simulink model "Simulador"  (R2015a)
settings: Solver=ode45  StartTime=0.0  StopTime=Inf  MaxStep=1  RelTol=1e-3
StopFcn:
  | close all
  | post_simulacion
model workspace (MAT data in the model file):
  m = 3.797
  b = 2.1
  c = 0.3571
  Salar = 0.75
  AR = 5.88
  cg = [0.44 0 0]
  Ix = 1.229
  Iy = 0.1702
  Iz = 0.8808
  Ixz = 0.9343
  e = 0.9935
  alpha0 = 0.267
  coefprop = [0.016415 -0.0142726]
  C_L0 = 0.0254
  C_Lalpha = 4.0191
  C_Lq = 3.8954
  C_Ldelta_e = 0.5872
  C_D0 = 0.0102
  C_Dbeta1 = -2.0864e-07
  C_Dbeta2 = 0.0671
  C_Dq = 0
  C_Ddelta_e = 0.8461
  C_Y0 = 3.2049e-18
  C_Ybeta = -0.1949
  C_Yp = -0.1172
  C_Yr = 0.0959
  C_Ydelta_a = -0.0696
  C_l0 = 1.1518e-18
  C_lbeta = -0.0765
  C_lp = -0.4018
  C_lr = 0.025
  C_ldelta_a = 0.2987
  C_m0 = 0.018
  C_malpha = -0.2524
  C_mq = -1.3047
  C_mdelta_e = -0.4857
  C_n0 = -2.2667e-07
  C_nbeta = 0.0403
  C_np = -0.0247
  C_nr = -0.1252
  C_ndelta_a = 0.0076
  gamma = 0.20958671
  gamma1 = 8.64638926772
  gamma2 = 7.15127867602
  gamma3 = 4.20255654569
  gamma4 = 4.4578208227
  gamma5 = -2.04582843713
  gamma6 = 5.48942420682
  gamma7 = 10.3736620037
  gamma8 = 5.86392142899
  C_p0 = -1.01045424588e-06
  C_pbeta = -0.14184539659
  C_pp = -1.79869539438
  C_pr = -0.45305525336
  C_pdelta_a = 1.28918307845
  C_r0 = -1.3291750703e-06
  C_rbeta = -0.104707259349
  C_rp = -1.93599126586
  C_rr = -0.622717442342
  C_rdelta_a = 1.3761168826
  C_mp = -0.2168
values from neighbouring files (symbols this model uses):
  r = [r_n;r_e;r_d]    [segmento.m]
  waypoints = reshape(waypoints_mat.',[],1)    [plan_de_vuelo.m]
undefined symbols (not defined in the file or in its folder): F, Light, magnitude, MIL, plan_de_vuelo
libraries: simulink_extras x20, aerolibconvert2 x18, aerolibfltsims x2, simulink x2, vrlib x1, instrumentlib x1, aerolibatmos2 x1, aerolibtransform2 x1, aerolibwind2 x1, aerolibgravity2 x1
(part 2 of 3)

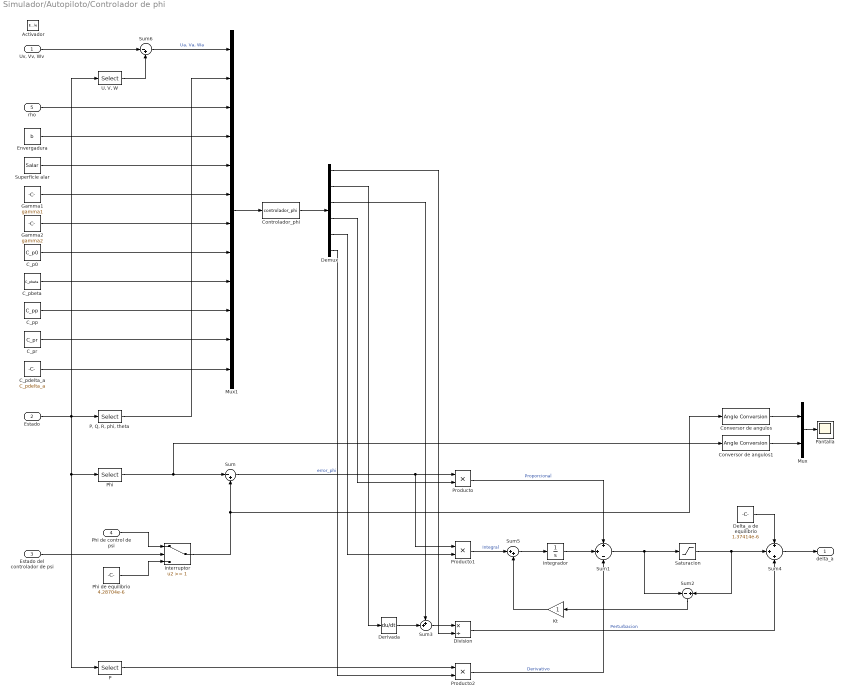
== system Simulador/Autopiloto/Controlador de phi ==
  "Uv, Vv, Wv" : Inport
  "Estado " : Inport  Port=2
  Estado del controlador de psi : Inport  Port=3  PortDimensions=1
  Phi de control de psi : Inport  Port=4  PortDimensions=1
  rho : Inport  Port=5
  Activador : EnablePort
  C_p0 : Constant  Value=C_p0
  C_pbeta : Constant  Value=C_pbeta
  C_pdelta_a : Constant  Value=C_pdelta_a
  C_pp : Constant  Value=C_pp
  C_pr : Constant  Value=C_pr
  Controlador_phi : MATLABFcn  MATLABFcn=controlador_phi  OutputDimensions=6
  Conversor de angulos : aerolibconvert2/Angle Conversion  IU=rad  OU=deg
  Conversor de angulos1 : aerolibconvert2/Angle Conversion  IU=rad  OU=deg
  Delta_a de equilibrio : Constant  Value=1.37414e-6
  Demux : Demux  Outputs=6
  Derivada : Derivative
  Division : Product  Inputs=*/
  Envergadura : Constant  Value=b
  Gamma1 : Constant  Value=gamma1
  Gamma2 : Constant  Value=gamma2
  Integrador : Integrator
  Interruptor : Switch  Threshold=1
  Kt : Gain
  Mux : Mux  Inputs=2
  Mux1 : Mux  Inputs=12
  P : Selector  InputPortWidth=12  Indices=4
      settings: AttributesFormatString=(Joystick - dependent)
  "P, Q, R, phi, theta" : Selector  InputPortWidth=12  Indices=[4 5 6 7 8]
      settings: AttributesFormatString=(Joystick - dependent)
  Pantalla : Scope
      settings: TimeRange=9.663330776874403  YMin=-35  YMax=50
  Phi : Selector  InputPortWidth=12  Indices=7
      settings: AttributesFormatString=(Joystick - dependent)
  Phi de equilibrio : Constant  Value=4.28704e-6
  Producto : Product
  Producto1 : Product
  Producto2 : Product
  Saturacion : Saturate  UpperLimit=5*pi/180  LowerLimit=-5*pi/180
  Sum : Sum  Inputs=|-+
  Sum1 : Sum  Inputs=+|+|-
  Sum2 : Sum  Inputs=-|+
  Sum3 : Sum  Inputs=++|
  Sum4 : Sum  Inputs=+|+|+
  Sum5 : Sum  Inputs=|++
  Sum6 : Sum  Inputs=|-+
  Superficie alar : Constant  Value=Salar
  "U, V, W" : Selector  InputPortWidth=12  Indices=[1 2 3]
      settings: AttributesFormatString=(Joystick - dependent)
  delta_a : Outport
  wires:
  "Estado "/1 -> "U, V, W"/1, P/1, Phi/1, "P, Q, R, phi, theta"/1
  Sum3/1 -> Division/1
  Phi/1 -> Conversor de angulos1/1, Sum/1
  Sum/1 -> Producto1/1, Producto/1  "error_phi"
  P/1 -> Producto2/1
  Producto2/1 -> Sum1/3  "Derivativo"
  Producto/1 -> Sum1/1  "Proporcional"
  Division/1 -> Sum4/3  "Perturbacion"
  Saturacion/1 -> Sum4/2, Sum2/2
  Producto1/1 -> Sum5/1  "Integral"
  Kt/1 -> Sum5/2
  Sum2/1 -> Kt/1
  Delta_a de equilibrio/1 -> Sum4/1
  Estado del controlador de psi/1 -> Interruptor/2
  Interruptor/1 -> Sum/2, Conversor de angulos/1
  Derivada/1 -> Sum3/2
  Sum1/1 -> Sum2/1, Saturacion/1
  Sum4/1 -> delta_a/1
  Integrador/1 -> Sum1/2
  Sum5/1 -> Integrador/1
  Mux1/1 -> Controlador_phi/1
  "U, V, W"/1 -> Sum6/2
  "Uv, Vv, Wv"/1 -> Sum6/1
  Sum6/1 -> Mux1/1  "Ua, Va, Wa"
  rho/1 -> Mux1/3
  "P, Q, R, phi, theta"/1 -> Mux1/2
  Mux/1 -> Pantalla/1
  Conversor de angulos/1 -> Mux/1
  Conversor de angulos1/1 -> Mux/2
  Phi de control de psi/1 -> Interruptor/1
  Phi de equilibrio/1 -> Interruptor/3
  Controlador_phi/1 -> Demux/1
  Demux/1 -> Division/2
  Demux/2 -> Derivada/1
  Demux/3 -> Sum3/1
  Demux/4 -> Producto/2
  Demux/5 -> Producto1/2
  Demux/6 -> Producto2/2
  Envergadura/1 -> Mux1/4
  Superficie alar/1 -> Mux1/5
  Gamma1/1 -> Mux1/6
  Gamma2/1 -> Mux1/7
  C_p0/1 -> Mux1/8
  C_pbeta/1 -> Mux1/9
  C_pp/1 -> Mux1/10
  C_pr/1 -> Mux1/11
  C_pdelta_a/1 -> Mux1/12

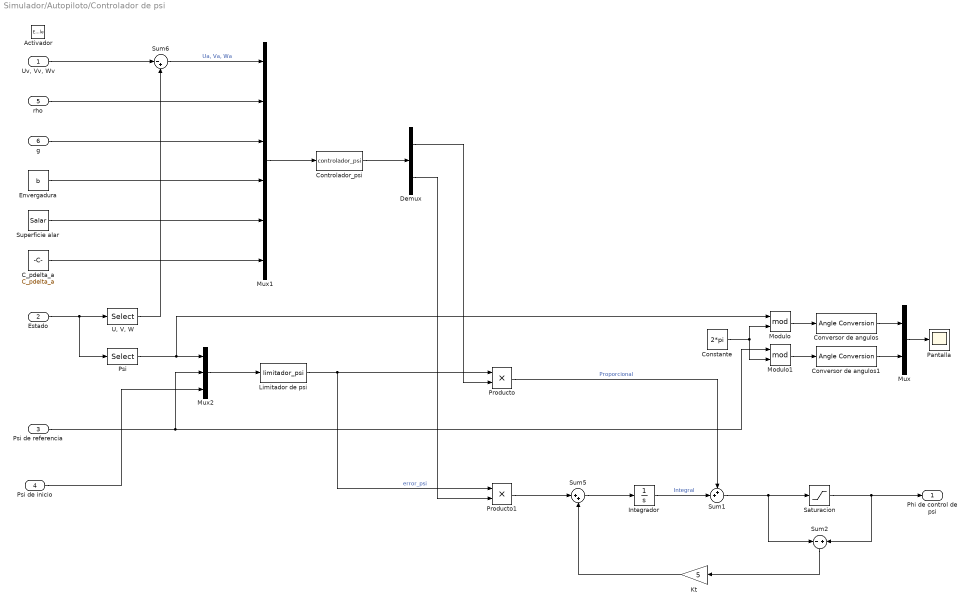
== system Simulador/Autopiloto/Controlador de psi ==
  "Uv, Vv, Wv" : Inport
  "Estado " : Inport  Port=2
  Psi de referencia : Inport  Port=3
  Psi de inicio : Inport  Port=4
  rho : Inport  Port=5
  g : Inport  Port=6
  Activador : EnablePort
  C_pdelta_a : Constant  Value=C_pdelta_a
  Constante : Constant  Value=2*pi
  Controlador_psi : MATLABFcn  MATLABFcn=controlador_psi  OutputDimensions=2
  Conversor de angulos : aerolibconvert2/Angle Conversion  IU=rad  OU=deg
  Conversor de angulos1 : aerolibconvert2/Angle Conversion  IU=rad  OU=deg
  Demux : Demux  Outputs=2
  Envergadura : Constant  Value=b
  Integrador : Integrator
  Kt : Gain  Gain=5
  Limitador de psi : MATLABFcn  MATLABFcn=limitador_psi  OutputDimensions=1
  Modulo : Math  Operator=mod  SaturateOnIntegerOverflow=on
  Modulo1 : Math  Operator=mod  SaturateOnIntegerOverflow=on
  Mux : Mux  Inputs=2
  Mux1 : Mux  Inputs=6
  Mux2 : Mux  Inputs=3
  Pantalla : Scope
      settings: TimeRange=9.663330776874403  YMin=0  YMax=450
  Producto : Product
  Producto1 : Product
  Psi : Selector  InputPortWidth=12  Indices=9
      settings: AttributesFormatString=(Joystick - dependent)
  Saturacion : Saturate  UpperLimit=30*pi/180  LowerLimit=-30*pi/180
  Sum1 : Sum  Inputs=++|
  Sum2 : Sum  Inputs=-|+
  Sum5 : Sum  Inputs=|++
  Sum6 : Sum  Inputs=|-+
  Superficie alar : Constant  Value=Salar
  "U, V, W" : Selector  InputPortWidth=12  Indices=[1 2 3]
      settings: AttributesFormatString=(Joystick - dependent)
  Phi de control de psi : Outport
  wires:
  "Estado "/1 -> "U, V, W"/1, Psi/1
  Controlador_psi/1 -> Demux/1
  Producto/1 -> Sum1/1  "Proporcional"
  Integrador/1 -> Sum1/2  "Integral"
  Kt/1 -> Sum5/2
  Sum2/1 -> Kt/1
  Sum1/1 -> Saturacion/1, Sum2/1
  Demux/2 -> Producto1/2
  Demux/1 -> Producto/2
  Producto1/1 -> Sum5/1
  Sum5/1 -> Integrador/1
  Mux1/1 -> Controlador_psi/1
  Saturacion/1 -> Phi de control de psi/1, Sum2/2
  Psi/1 -> Modulo/1, Mux2/1
  Psi de referencia/1 -> Modulo1/1, Mux2/2
  Mux2/1 -> Limitador de psi/1
  Limitador de psi/1 -> Producto1/1, Producto/1  "error_psi"
  "U, V, W"/1 -> Sum6/2
  "Uv, Vv, Wv"/1 -> Sum6/1
  Sum6/1 -> Mux1/1  "Ua, Va, Wa"
  Mux/1 -> Pantalla/1
  Conversor de angulos/1 -> Mux/1
  Conversor de angulos1/1 -> Mux/2
  Modulo1/1 -> Conversor de angulos1/1
  Modulo/1 -> Conversor de angulos/1
  Constante/1 -> Modulo/2, Modulo1/2
  rho/1 -> Mux1/2
  Psi de inicio/1 -> Mux2/3
  g/1 -> Mux1/3
  C_pdelta_a/1 -> Mux1/6
  Superficie alar/1 -> Mux1/5
  Envergadura/1 -> Mux1/4

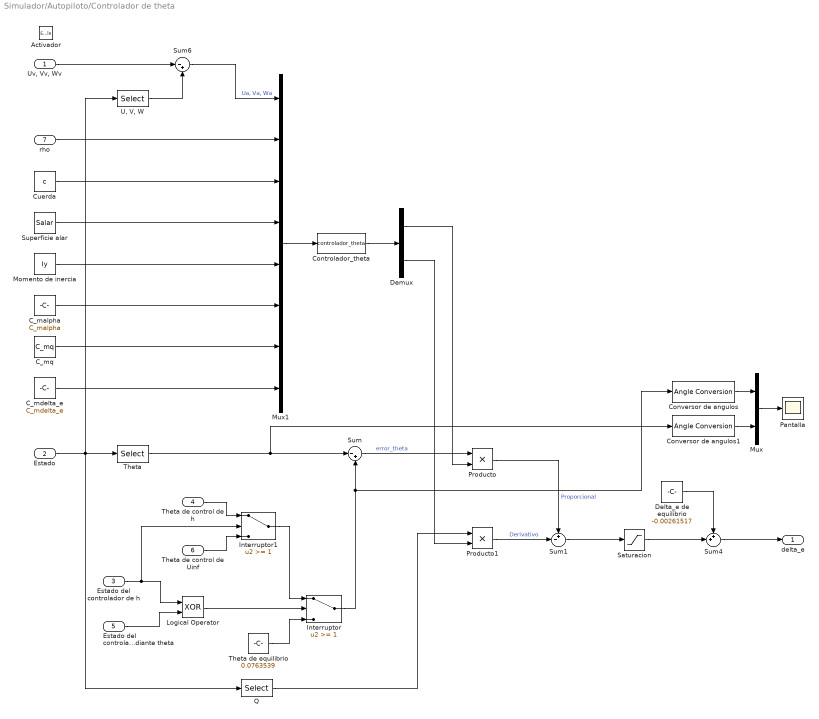
== system Simulador/Autopiloto/Controlador de theta ==
  "Uv, Vv, Wv" : Inport
  "Estado " : Inport  Port=2
  Estado del controlador de h : Inport  Port=3
  Theta de control de h : Inport  Port=4
  Estado del controlador de Uinf mediante theta : Inport  Port=5
  Theta de control de Uinf : Inport  Port=6
  rho : Inport  Port=7
  Activador : EnablePort
  C_malpha : Constant  Value=C_malpha
  C_mdelta_e : Constant  Value=C_mdelta_e
  C_mq : Constant  Value=C_mq
  Controlador_theta : MATLABFcn  MATLABFcn=controlador_theta  OutputDimensions=2
  Conversor de angulos : aerolibconvert2/Angle Conversion  IU=rad  OU=deg
  Conversor de angulos1 : aerolibconvert2/Angle Conversion  IU=rad  OU=deg
  Cuerda : Constant  Value=c
  Delta_e de equilibrio : Constant  Value=-0.00261517
  Demux : Demux  Outputs=2
  Interruptor : Switch  Threshold=1
  Interruptor1 : Switch  Threshold=1
  Logical Operator : Logic  Operator=XOR  AllPortsSameDT=off  OutDataTypeStr=boolean
  Momento de inercia : Constant  Value=Iy
  Mux : Mux  Inputs=2
  Mux1 : Mux  Inputs=8
  Pantalla : Scope
      settings: TimeRange=9.663330776874403  YMax=20  SaveName=ScopeData4
  Producto : Product
  Producto1 : Product
  Q : Selector  InputPortWidth=12  Indices=5
      settings: AttributesFormatString=(Joystick - dependent)
  Saturacion : Saturate  UpperLimit=5*pi/180  LowerLimit=-5*pi/180
  Sum : Sum  Inputs=|-+
  Sum1 : Sum  Inputs=+-|
  Sum4 : Sum  Inputs=++|
  Sum6 : Sum  Inputs=|-+
  Superficie alar : Constant  Value=Salar
  Theta : Selector  InputPortWidth=12  Indices=8
      settings: AttributesFormatString=(Joystick - dependent)
  Theta de equilibrio : Constant  Value=0.0763539
  "U, V, W" : Selector  InputPortWidth=12  Indices=[1 2 3]
      settings: AttributesFormatString=(Joystick - dependent)
  delta_e : Outport
  wires:
  Controlador_theta/1 -> Demux/1
  Theta/1 -> Conversor de angulos1/1, Sum/1
  Sum/1 -> Producto/1  "error_theta"
  Producto/1 -> Sum1/1  "Proporcional"
  Producto1/1 -> Sum1/2  "Derivativo"
  Sum1/1 -> Saturacion/1
  Sum4/1 -> delta_e/1
  Demux/1 -> Producto/2
  Q/1 -> Producto1/1
  Demux/2 -> Producto1/2
  Delta_e de equilibrio/1 -> Sum4/1
  Theta de equilibrio/1 -> Interruptor/3
  Interruptor/1 -> Conversor de angulos/1, Sum/2
  Estado del controlador de h/1 -> Logical Operator/1, Interruptor1/2
  Estado del controlador de Uinf mediante theta/1 -> Logical Operator/2
  Logical Operator/1 -> Interruptor/2
  Theta de control de h/1 -> Interruptor1/1
  Interruptor1/1 -> Interruptor/1
  Saturacion/1 -> Sum4/2
  Mux/1 -> Pantalla/1
  Conversor de angulos/1 -> Mux/1
  Conversor de angulos1/1 -> Mux/2
  "Estado "/1 -> Q/1, "U, V, W"/1, Theta/1
  "U, V, W"/1 -> Sum6/2
  "Uv, Vv, Wv"/1 -> Sum6/1
  Theta de control de Uinf/1 -> Interruptor1/3
  Mux1/1 -> Controlador_theta/1
  Sum6/1 -> Mux1/1  "Ua, Va, Wa"
  rho/1 -> Mux1/2
  Cuerda/1 -> Mux1/3
  Superficie alar/1 -> Mux1/4
  Momento de inercia/1 -> Mux1/5
  C_malpha/1 -> Mux1/6
  C_mq/1 -> Mux1/7
  C_mdelta_e/1 -> Mux1/8

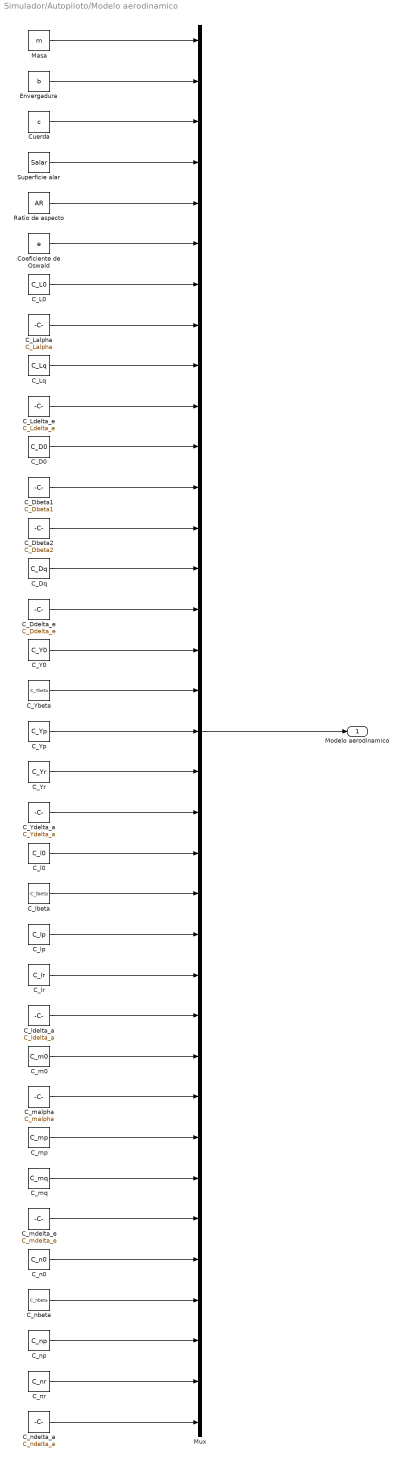
== system Simulador/Autopiloto/Modelo aerodinamico ==
  C_D0 : Constant  Value=C_D0
  C_Dbeta1 : Constant  Value=C_Dbeta1
  C_Dbeta2 : Constant  Value=C_Dbeta2
  C_Ddelta_e : Constant  Value=C_Ddelta_e
  C_Dq : Constant  Value=C_Dq
  C_L0 : Constant  Value=C_L0
  C_Lalpha : Constant  Value=C_Lalpha
  C_Ldelta_e : Constant  Value=C_Ldelta_e
  C_Lq : Constant  Value=C_Lq
  C_Y0 : Constant  Value=C_Y0
  C_Ybeta : Constant  Value=C_Ybeta
  C_Ydelta_a : Constant  Value=C_Ydelta_a
  C_Yp : Constant  Value=C_Yp
  C_Yr : Constant  Value=C_Yr
  C_l0 : Constant  Value=C_l0
  C_lbeta : Constant  Value=C_lbeta
  C_ldelta_a : Constant  Value=C_ldelta_a
  C_lp : Constant  Value=C_lp
  C_lr : Constant  Value=C_lr
  C_m0 : Constant  Value=C_m0
  C_malpha : Constant  Value=C_malpha
  C_mdelta_e : Constant  Value=C_mdelta_e
  C_mp : Constant  Value=C_mp
  C_mq : Constant  Value=C_mq
  C_n0 : Constant  Value=C_n0
  C_nbeta : Constant  Value=C_nbeta
  C_ndelta_a : Constant  Value=C_ndelta_a
  C_np : Constant  Value=C_np
  C_nr : Constant  Value=C_nr
  Coeficiente de Oswald : Constant  Value=e
  Cuerda : Constant  Value=c
  Envergadura : Constant  Value=b
  Masa : Constant  Value=m
  Mux : Mux  Inputs=35
  Ratio de aspecto : Constant  Value=AR
  Superficie alar : Constant  Value=Salar
  Modelo aerodinamico : Outport
  wires:
  Mux/1 -> Modelo aerodinamico/1
  C_ndelta_a/1 -> Mux/35
  C_nr/1 -> Mux/34
  C_np/1 -> Mux/33
  C_nbeta/1 -> Mux/32
  C_n0/1 -> Mux/31
  C_mdelta_e/1 -> Mux/30
  C_mq/1 -> Mux/29
  C_mp/1 -> Mux/28
  C_malpha/1 -> Mux/27
  C_m0/1 -> Mux/26
  C_ldelta_a/1 -> Mux/25
  C_lr/1 -> Mux/24
  C_lp/1 -> Mux/23
  C_lbeta/1 -> Mux/22
  C_l0/1 -> Mux/21
  C_Ydelta_a/1 -> Mux/20
  C_Yr/1 -> Mux/19
  C_Yp/1 -> Mux/18
  C_Ybeta/1 -> Mux/17
  C_Y0/1 -> Mux/16
  C_Ddelta_e/1 -> Mux/15
  C_Dq/1 -> Mux/14
  C_Dbeta2/1 -> Mux/13
  C_Dbeta1/1 -> Mux/12
  C_D0/1 -> Mux/11
  C_Ldelta_e/1 -> Mux/10
  C_Lq/1 -> Mux/9
  C_Lalpha/1 -> Mux/8
  C_L0/1 -> Mux/7
  Masa/1 -> Mux/1
  Envergadura/1 -> Mux/2
  Cuerda/1 -> Mux/3
  Superficie alar/1 -> Mux/4
  Ratio de aspecto/1 -> Mux/5
  Coeficiente de Oswald/1 -> Mux/6

== system Simulador/Autopiloto/Reconocedor de inicio del controlador de psi ==
  Estado del controlador de psi (manual) : Inport
  Psi (manual) : Inport  Port=2
  Estado del controlador de psi (FMS) : Inport  Port=3
  Tramo (FMS) : Inport  Port=4
  Psi : Inport  Port=5
  Constante : Constant  OutDataTypeStr=boolean
  Constante1 : Constant  OutDataTypeStr=boolean
  Conversor de tipologia de datos : DataTypeConversion  OutDataTypeStr=boolean
  Conversor de tipologia de datos1 : DataTypeConversion  OutDataTypeStr=double
  Detector de subida : simulink/Logic and Bit Operations/Detect Increase  vinit=0.0  InputProcessing=Inherited  OutDataTypeStr=boolean
  Interruptor : Switch  Criteria=u2 ~= 0
  Interruptor1 : Switch  Criteria=u2 ~= 0
  Interruptor2 : Switch  Criteria=u2 > Threshold
  Interruptor3 : Switch  Criteria=u2 ~= 0
  Memoria : Memory
  Memoria1 : Memory
  Operador logico : Logic  Operator=OR  Inputs=3  AllPortsSameDT=off  OutDataTypeStr=boolean
  Operador logico1 : Logic  AllPortsSameDT=off  OutDataTypeStr=boolean
  Psi de inicio : Subsystem
  Sum : Sum  Inputs=|+-
  Sum1 : Sum  Inputs=|+-
  Tierra : Ground
  Tierra1 : Ground
  Psi_inicio_ : Outport
  wires:
  Estado del controlador de psi (manual)/1 -> Conversor de tipologia de datos/1
  Conversor de tipologia de datos/1 -> Detector de subida/1
  Conversor de tipologia de datos1/1 -> Psi de inicio/Trigger
  Memoria/1 -> Sum/2
  Psi (manual)/1 -> Memoria/1, Sum/1
  Sum/1 -> Interruptor/2
  Tierra/1 -> Interruptor/3
  Constante/1 -> Interruptor/1
  Operador logico/1 -> Conversor de tipologia de datos1/1
  Memoria1/1 -> Sum1/2
  Sum1/1 -> Interruptor1/2
  Tierra1/1 -> Interruptor1/3
  Constante1/1 -> Interruptor1/1
  Interruptor1/1 -> Operador logico1/2
  Estado del controlador de psi (FMS)/1 -> Operador logico1/1, Interruptor3/2
  Operador logico1/1 -> Operador logico/3
  Interruptor/1 -> Operador logico/2
  Detector de subida/1 -> Operador logico/1
  Psi/1 -> Interruptor2/3, Psi de inicio/1(Psi)
  Tramo (FMS)/1 -> Interruptor2/2, Memoria1/1, Sum1/1
  Interruptor2/1 -> Interruptor3/1
  Interruptor3/1 -> Psi_inicio_/1
  Psi de inicio/1(Psi_) -> Interruptor3/3, Interruptor2/1

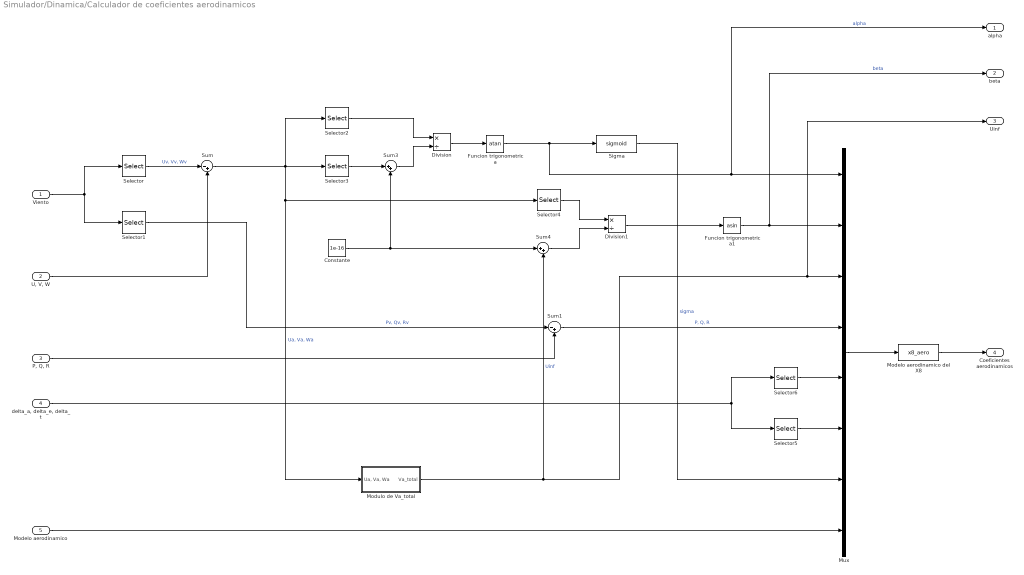
== system Simulador/Dinamica/Calculador de coeficientes aerodinamicos ==
  Viento : Inport
  "U, V, W" : Inport  Port=2
  "P, Q, R" : Inport  Port=3
  "delta_a, delta_e, delta_t" : Inport  Port=4
  Modelo aerodinamico : Inport  Port=5
  Constante : Constant  Value=1e-16
  Division : Product  Inputs=*/
  Division1 : Product  Inputs=*/
  Funcion trigonometrica : Trigonometry  Operator=atan
  Funcion trigonometrica1 : Trigonometry  Operator=asin
  Modelo aerodinamico del X8 : MATLABFcn  MATLABFcn=x8_aero  OutputDimensions=6
  Modulo de Va_total : Subsystem
  Mux : Mux  Inputs=8
  Selector : Selector  InputPortWidth=6  Indices=[1 2 3]
  Selector1 : Selector  InputPortWidth=6  Indices=[4 5 6]
  Selector2 : Selector  InputPortWidth=3  Indices=3
  Selector3 : Selector  InputPortWidth=3
  Selector4 : Selector  InputPortWidth=3  Indices=2
  Selector5 : Selector  InputPortWidth=3  Indices=2
  Selector6 : Selector  InputPortWidth=3
  Sigma : MATLABFcn  MATLABFcn=sigmoid  OutputDimensions=1
  Sum : Sum  Inputs=|-+
  Sum1 : Sum  Inputs=|-+
  Sum3 : Sum  Inputs=|++
  Sum4 : Sum  Inputs=|++
  alpha : Outport
  beta : Outport  Port=2
  Uinf : Outport  Port=3
  Coeficientes aerodinamicos : Outport  Port=4
  wires:
  Viento/1 -> Selector/1, Selector1/1
  "U, V, W"/1 -> Sum/2
  Selector/1 -> Sum/1  "Uv, Vv, Wv"
  Selector1/1 -> Sum1/1  "Pv, Qv, Rv"
  "P, Q, R"/1 -> Sum1/2
  Sum/1 -> Selector3/1, Selector2/1, Selector4/1, Modulo de Va_total/1("Ua, Va, Wa")  "Ua, Va, Wa"
  Selector2/1 -> Division/1
  Sum3/1 -> Division/2
  Division/1 -> Funcion trigonometrica/1
  Division1/1 -> Funcion trigonometrica1/1
  Selector4/1 -> Division1/1
  Sum4/1 -> Division1/2
  Modulo de Va_total/1(Va_total) -> Uinf/1, Mux/3, Sum4/2  "Uinf"
  Funcion trigonometrica/1 -> Sigma/1, alpha/1, Mux/1  "alpha"
  Funcion trigonometrica1/1 -> Mux/2, beta/1  "beta"
  "delta_a, delta_e, delta_t"/1 -> Selector5/1, Selector6/1
  Mux/1 -> Modelo aerodinamico del X8/1
  Modelo aerodinamico del X8/1 -> Coeficientes aerodinamicos/1
  Constante/1 -> Sum4/1, Sum3/2
  Selector3/1 -> Sum3/1
  Sum1/1 -> Mux/4  "P, Q, R"
  Selector5/1 -> Mux/6
  Selector6/1 -> Mux/5
  Sigma/1 -> Mux/7  "sigma"
  Modelo aerodinamico/1 -> Mux/8

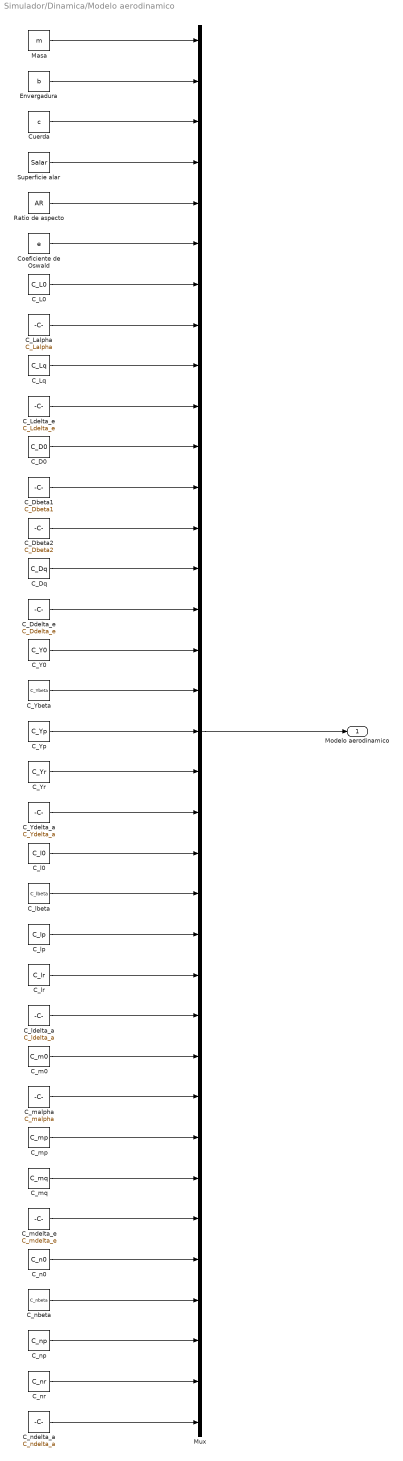
== system Simulador/Dinamica/Modelo aerodinamico ==
  C_D0 : Constant  Value=C_D0
  C_Dbeta1 : Constant  Value=C_Dbeta1
  C_Dbeta2 : Constant  Value=C_Dbeta2
  C_Ddelta_e : Constant  Value=C_Ddelta_e
  C_Dq : Constant  Value=C_Dq
  C_L0 : Constant  Value=C_L0
  C_Lalpha : Constant  Value=C_Lalpha
  C_Ldelta_e : Constant  Value=C_Ldelta_e
  C_Lq : Constant  Value=C_Lq
  C_Y0 : Constant  Value=C_Y0
  C_Ybeta : Constant  Value=C_Ybeta
  C_Ydelta_a : Constant  Value=C_Ydelta_a
  C_Yp : Constant  Value=C_Yp
  C_Yr : Constant  Value=C_Yr
  C_l0 : Constant  Value=C_l0
  C_lbeta : Constant  Value=C_lbeta
  C_ldelta_a : Constant  Value=C_ldelta_a
  C_lp : Constant  Value=C_lp
  C_lr : Constant  Value=C_lr
  C_m0 : Constant  Value=C_m0
  C_malpha : Constant  Value=C_malpha
  C_mdelta_e : Constant  Value=C_mdelta_e
  C_mp : Constant  Value=C_mp
  C_mq : Constant  Value=C_mq
  C_n0 : Constant  Value=C_n0
  C_nbeta : Constant  Value=C_nbeta
  C_ndelta_a : Constant  Value=C_ndelta_a
  C_np : Constant  Value=C_np
  C_nr : Constant  Value=C_nr
  Coeficiente de Oswald : Constant  Value=e
  Cuerda : Constant  Value=c
  Envergadura : Constant  Value=b
  Masa : Constant  Value=m
  Mux : Mux  Inputs=35
  Ratio de aspecto : Constant  Value=AR
  Superficie alar : Constant  Value=Salar
  Modelo aerodinamico : Outport
  wires:
  Mux/1 -> Modelo aerodinamico/1
  C_ndelta_a/1 -> Mux/35
  C_nr/1 -> Mux/34
  C_np/1 -> Mux/33
  C_nbeta/1 -> Mux/32
  C_n0/1 -> Mux/31
  C_mdelta_e/1 -> Mux/30
  C_mq/1 -> Mux/29
  C_mp/1 -> Mux/28
  C_malpha/1 -> Mux/27
  C_m0/1 -> Mux/26
  C_ldelta_a/1 -> Mux/25
  C_lr/1 -> Mux/24
  C_lp/1 -> Mux/23
  C_lbeta/1 -> Mux/22
  C_l0/1 -> Mux/21
  C_Ydelta_a/1 -> Mux/20
  C_Yr/1 -> Mux/19
  C_Yp/1 -> Mux/18
  C_Ybeta/1 -> Mux/17
  C_Y0/1 -> Mux/16
  C_Ddelta_e/1 -> Mux/15
  C_Dq/1 -> Mux/14
  C_Dbeta2/1 -> Mux/13
  C_Dbeta1/1 -> Mux/12
  C_D0/1 -> Mux/11
  C_Ldelta_e/1 -> Mux/10
  C_Lq/1 -> Mux/9
  C_Lalpha/1 -> Mux/8
  C_L0/1 -> Mux/7
  Masa/1 -> Mux/1
  Envergadura/1 -> Mux/2
  Cuerda/1 -> Mux/3
  Superficie alar/1 -> Mux/4
  Ratio de aspecto/1 -> Mux/5
  Coeficiente de Oswald/1 -> Mux/6

== system Simulador/Entrada de control manual/Palanca de mando ==
  Activador : EnablePort
  Palanca de mando : vrlib/Joystick Input  joyid=2  adjustports=on  forcefeed=off
  Selector de botones : Selector  InputPortWidth=11  Indices=[1 2 3 4 5 6 7 8 9 10 11]
      settings: AttributesFormatString=(Joystick - dependent)
  Selector de ejes : Selector  InputPortWidth=3  Indices=[1 2 3]
      settings: AttributesFormatString=(Joystick - dependent)
  Ejes : Outport
  Botones : Outport  Port=2
  wires:
  Palanca de mando/2 -> Selector de botones/1
  Selector de botones/1 -> Botones/1
  Palanca de mando/1 -> Selector de ejes/1
  Selector de ejes/1 -> Ejes/1

== system Simulador/Entrada de control manual/Teclado ==
  Activador : EnablePort
  Constante : Constant  Value=0
  Conversor de tipologia de datos : DataTypeConversion  OutDataTypeStr=boolean
  Memoria : Memory
  Reconocedor de teclado : Subsystem  TreatAsAtomicUnit=on
  Sum1 : Sum  Inputs=++|
  Teclado : M-S-Function  FunctionName=sfun_keyboard_input_v1_2b  mask(Keyboard Input){}
      mask help: Keyboard Input
      mask Display: fprintf('Keyboard');
  Ejes : Outport  PortDimensions=3
  Botones : Outport  Port=2  PortDimensions=11
  wires:
  Teclado/1 -> Reconocedor de teclado/1(Tecla)
  Teclado/2 -> Conversor de tipologia de datos/1
  Sum1/1 -> Reconocedor de teclado/2(Ejes)
  Constante/1 -> Sum1/1
  Reconocedor de teclado/1(Ejes_) -> Ejes/1, Memoria/1
  Memoria/1 -> Sum1/2
  Reconocedor de teclado/2(Botones_) -> Botones/1
  Conversor de tipologia de datos/1 -> Reconocedor de teclado/Enable, Reconocedor de teclado/3(Pulsacion)

== system Simulador/Leyes de actuacion/Ley de alerones ==
  Alerones PWM : Inport
  Constante : Constant  Value=2*(2100-1520)
  Conversor de angulos : aerolibconvert2/Angle Conversion  IU=deg  OU=rad
  Division : Product  Inputs=*/
  PWM_0 : Constant  Value=1520
  Rango angular : Gain  Gain=10
  Saturacion : Saturate  UpperLimit=5  LowerLimit=-5
  Sum1 : Sum  Inputs=|+-
  delta_a : Outport
  wires:
  Alerones PWM/1 -> Sum1/1
  PWM_0/1 -> Sum1/2
  Sum1/1 -> Rango angular/1
  Rango angular/1 -> Division/1
  Constante/1 -> Division/2
  Division/1 -> Saturacion/1
  Conversor de angulos/1 -> delta_a/1
  Saturacion/1 -> Conversor de angulos/1

== system Simulador/Leyes de actuacion/Ley de elevadores ==
  Elevadores PWM : Inport
  Constante : Constant  Value=2*(2100-1520)
  Conversor de angulos : aerolibconvert2/Angle Conversion  IU=deg  OU=rad
  Division : Product  Inputs=*/
  Inversion : Gain  Gain=-1
  PWM_0 : Constant  Value=1520
  Rango angular : Gain  Gain=30
  Saturacion : Saturate  UpperLimit=15  LowerLimit=-15
  Sum1 : Sum  Inputs=|+-
  delta_e : Outport
  wires:
  PWM_0/1 -> Sum1/2
  Sum1/1 -> Rango angular/1
  Rango angular/1 -> Division/1
  Constante/1 -> Division/2
  Conversor de angulos/1 -> delta_e/1
  Saturacion/1 -> Conversor de angulos/1
  Elevadores PWM/1 -> Sum1/1
  Division/1 -> Inversion/1
  Inversion/1 -> Saturacion/1

== system Simulador/Leyes de actuacion/Ley de propulsion ==
  Motor PWM : Inport
  Ua : Inport  Port=2
  Coefprop_U^2 : Gain  Gain=coefprop(2)
  Coefprop_motor_pwm : Gain  Gain=coefprop(1)
  PWM_1 : Constant  Value=1100
  Producto : Product  Inputs=**
  Sum : Sum
  Sum1 : Sum  Inputs=|+-
  delta_t : Outport
  wires:
  Ua/1 -> Producto/2, Producto/1
  Motor PWM/1 -> Sum1/1
  PWM_1/1 -> Sum1/2
  Sum1/1 -> Coefprop_motor_pwm/1
  Producto/1 -> Coefprop_U^2/1
  Sum/1 -> delta_t/1
  Coefprop_U^2/1 -> Sum/2
  Coefprop_motor_pwm/1 -> Sum/1

== system Simulador/Mision/Gestor de GPS ==
  Posicion_geodetica : Inport
  "Psi " : Inport  Port=2  SampleTime=1
  Activador : EnablePort
  Constante : Constant  Value=2
  Constante1 : Constant
  Envio de datos : Subsystem  TreatAsAtomicUnit=on
  Interruptor : Switch  Criteria=u2 ~= 0
  Mux : Mux  Inputs=3
  Reloj : DigitalClock
  Remanente : Math  Operator=rem  SaturateOnIntegerOverflow=on
  Selector : Selector  InputPortWidth=3  Indices=[1 2]
  Tierra : Ground
  wires:
  Reloj/1 -> Mux/3, Remanente/1
  Selector/1 -> Mux/1
  Constante/1 -> Remanente/2
  Remanente/1 -> Interruptor/2
  Constante1/1 -> Interruptor/3
  Tierra/1 -> Interruptor/1
  Interruptor/1 -> Envio de datos/Enable
  Mux/1 -> Envio de datos/1(Datos)
  "Psi "/1 -> Mux/2
  Posicion_geodetica/1 -> Selector/1

== system Simulador/Mision/Gestor de trayectorias ==
  Posicion_NED : Inport
  Posicion_geodetica_inicial : Inport  Port=2
  Psi : Inport  Port=3
  Posicion_NED_reinicio : Inport  Port=4
  Reinicio_disparador : Inport  Port=5
  Activador : EnablePort
  Demux : Demux  Outputs=2
  Geodeticas a NED : MATLABFcn  MATLABFcn=geodeticas_ned_mat  Output1D=off
  Memoria : Memory  X0=1
  Memoria1 : Memory  X0=1
  Mux : Mux  Inputs=3
  Mux1 : Mux
  Mux2 : Mux  Inputs=5
  Mux3 : Mux  Inputs=2
  Plan de vuelo : Constant  Value=waypoints
  Ruta : MATLABFcn  MATLABFcn=ruta  OutputDimensions=7
  Segmento : MATLABFcn  MATLABFcn=segmento  OutputDimensions=2
  Selector : Selector  InputPortWidth=7  Indices=[1 2 3]
  Selector1 : Selector  InputPortWidth=7  Indices=[4 5 6]
  Selector2 : Selector  InputPortWidth=7  Indices=7
  Selector3 : Selector  InputPortWidth=3  Indices=3
  Sum : Sum  Inputs=|++
  Valor inicial : InitialCondition  Value=2
  FMS_AP : Outport
  wires:
  Posicion_NED/1 -> Mux1/1, Mux2/3
  Mux2/1 -> Ruta/1
  Psi/1 -> Mux1/4
  Mux1/1 -> Segmento/1
  Ruta/1 -> Selector1/1, Selector/1, Selector2/1
  Selector/1 -> Mux1/2
  Selector1/1 -> Mux1/3
  Posicion_geodetica_inicial/1 -> Mux3/1, Selector3/1
  Demux/1 -> Mux/1
  Mux/1 -> FMS_AP/1
  Segmento/1 -> Demux/1
  Demux/2 -> Sum/1
  Sum/1 -> Mux/2
  Selector3/1 -> Sum/2
  Selector2/1 -> Mux/3, Memoria/1  "Tramo"
  Reinicio_disparador/1 -> Memoria1/1
  Valor inicial/1 -> Mux2/1
  Plan de vuelo/1 -> Mux3/2
  Mux3/1 -> Geodeticas a NED/1
  Geodeticas a NED/1 -> Mux2/5
  Posicion_NED_reinicio/1 -> Mux2/2
  Memoria/1 -> Mux2/4
  Memoria1/1 -> Valor inicial/1

== system Simulador/Mision/Reconocedor de reinicio de FMS ==
  FMS : Inport
  Posicion_NED : Inport  Port=2
  Conversor de tipologia de datos : DataTypeConversion  OutDataTypeStr=boolean
  Conversor de tipologia de datos1 : DataTypeConversion  OutDataTypeStr=double
  Detector de subida : simulink/Logic and Bit Operations/Detect Increase  vinit=0.0  InputProcessing=Inherited  OutDataTypeStr=boolean
  Posicion_NED de reinicio : Subsystem
  Disparo : Outport
  Posicion_NED_reinicio : Outport  Port=2
  wires:
  Posicion_NED/1 -> Posicion_NED de reinicio/1(Posicion_NED)
  Posicion_NED de reinicio/1(Posicion_NED_) -> Posicion_NED_reinicio/1
  FMS/1 -> Conversor de tipologia de datos/1, Posicion_NED de reinicio/Trigger
  Detector de subida/1 -> Conversor de tipologia de datos1/1
  Conversor de tipologia de datos/1 -> Detector de subida/1
  Conversor de tipologia de datos1/1 -> Disparo/1

== system Simulador/Modelo de viento/Modulo de V_total ==
  "U, V, W" : Inport
  Al cuadrado : Math  Operator=magnitude^2  SaturateOnIntegerOverflow=on
  Al cuadrado1 : Math  Operator=magnitude^2  SaturateOnIntegerOverflow=on
  Al cuadrado2 : Math  Operator=magnitude^2  SaturateOnIntegerOverflow=on
  Demux1 : Demux  Outputs=3
  Raiz cuadrada : Sqrt  SaturateOnIntegerOverflow=on
  Sum2 : Sum  Inputs=+++
  V_total : Outport
  wires:
  "U, V, W"/1 -> Demux1/1
  Demux1/2 -> Al cuadrado1/1
  Demux1/1 -> Al cuadrado/1
  Demux1/3 -> Al cuadrado2/1
  Al cuadrado1/1 -> Sum2/2
  Al cuadrado2/1 -> Sum2/3
  Al cuadrado/1 -> Sum2/1
  Sum2/1 -> Raiz cuadrada/1
  Raiz cuadrada/1 -> V_total/1

== system Simulador/Modelo de viento/Subsistema de modelo de viento ==
  Altitud : Inport
  V_total : Inport  Port=2
  R_bn : Inport  Port=3
  Activador : EnablePort
  Modelo Dryden de viento (Continuo (+q +r)) : aerolibwind2/Dryden Wind Turbulence Model  (Continuous (+q -r))  units=Metric (MKS)  spec=MIL-F-8785C  model=Continuous Dryden (+q +r)  W20=15  Wdeg=225  TurbProb=10^-2 - Light  L_high=533.4  Wingspan=2.1  ts=0.1  Seed=[23341 23342 23343 23344]  T_on=on
  V_viento : Outport
  W_viento : Outport  Port=2
  wires:
  Altitud/1 -> Modelo Dryden de viento (Continuo (+q +r))/1
  V_total/1 -> Modelo Dryden de viento (Continuo (+q +r))/2
  R_bn/1 -> Modelo Dryden de viento (Continuo (+q +r))/3
  Modelo Dryden de viento (Continuo (+q +r))/1 -> V_viento/1
  Modelo Dryden de viento (Continuo (+q +r))/2 -> W_viento/1

== system Simulador/Pre visualizacion/Modulo de Va_total ==
  "Ua, Va, Wa" : Inport
  Al cuadrado : Math  Operator=magnitude^2  SaturateOnIntegerOverflow=on
  Al cuadrado1 : Math  Operator=magnitude^2  SaturateOnIntegerOverflow=on
  Al cuadrado2 : Math  Operator=magnitude^2  SaturateOnIntegerOverflow=on
  Demux1 : Demux  Outputs=3
  Raiz cuadrada : Sqrt  SaturateOnIntegerOverflow=on
  Sum2 : Sum  Inputs=+++
  Va_total : Outport
  wires:
  "Ua, Va, Wa"/1 -> Demux1/1
  Demux1/2 -> Al cuadrado1/1
  Demux1/1 -> Al cuadrado/1
  Demux1/3 -> Al cuadrado2/1
  Al cuadrado1/1 -> Sum2/2
  Al cuadrado2/1 -> Sum2/3
  Al cuadrado/1 -> Sum2/1
  Sum2/1 -> Raiz cuadrada/1
  Raiz cuadrada/1 -> Va_total/1

== system Simulador/Autopiloto/Activador de controladores/Interruptor con latch ==
  Estado del boton : Inport
  Reinicio : Inport  Port=2
  Memoria de pulsacion del joystick : Subsystem  TreatAsAtomicUnit=on
  Memoria de pulsacion del teclado : Subsystem  TreatAsAtomicUnit=on
  Operador logico : Logic  Operator=NOT  AllPortsSameDT=off  OutDataTypeStr=boolean
  Operador logico1 : Logic  Operator=OR  AllPortsSameDT=off  OutDataTypeStr=boolean
  Estado del controlador : Outport
  wires:
  [Entrada] -> Operador logico/1, Memoria de pulsacion del joystick/Enable
  Estado del boton/1 -> Memoria de pulsacion del teclado/1(Estado del boton), Memoria de pulsacion del joystick/1(Estado del boton)
  Reinicio/1 -> Memoria de pulsacion del teclado/2(Reinicio), Memoria de pulsacion del joystick/2(Reinicio)
  Operador logico/1 -> Memoria de pulsacion del teclado/Enable
  Memoria de pulsacion del joystick/1(Estado del controlador) -> Operador logico1/1
  Memoria de pulsacion del teclado/1(Estado del controlador) -> Operador logico1/2
  Operador logico1/1 -> Estado del controlador/1

== system Simulador/Autopiloto/Activador de controladores/Interruptor con latch1 ==
  Estado del boton : Inport
  Reinicio : Inport  Port=2
  Memoria de pulsacion del joystick : Subsystem  TreatAsAtomicUnit=on
  Memoria de pulsacion del teclado : Subsystem  TreatAsAtomicUnit=on
  Operador logico : Logic  Operator=NOT  AllPortsSameDT=off  OutDataTypeStr=boolean
  Operador logico1 : Logic  Operator=OR  AllPortsSameDT=off  OutDataTypeStr=boolean
  Estado del controlador : Outport
  wires:
  [Entrada] -> Operador logico/1, Memoria de pulsacion del joystick/Enable
  Estado del boton/1 -> Memoria de pulsacion del teclado/1(Estado del boton), Memoria de pulsacion del joystick/1(Estado del boton)
  Reinicio/1 -> Memoria de pulsacion del teclado/2(Reinicio), Memoria de pulsacion del joystick/2(Reinicio)
  Operador logico/1 -> Memoria de pulsacion del teclado/Enable
  Memoria de pulsacion del joystick/1(Estado del controlador) -> Operador logico1/1
  Memoria de pulsacion del teclado/1(Estado del controlador) -> Operador logico1/2
  Operador logico1/1 -> Estado del controlador/1

== system Simulador/Autopiloto/Activador de controladores/Interruptor con latch2 ==
  Estado del boton : Inport
  Reinicio : Inport  Port=2
  Memoria de pulsacion del joystick : Subsystem  TreatAsAtomicUnit=on
  Memoria de pulsacion del teclado : Subsystem  TreatAsAtomicUnit=on
  Operador logico : Logic  Operator=NOT  AllPortsSameDT=off  OutDataTypeStr=boolean
  Operador logico1 : Logic  Operator=OR  AllPortsSameDT=off  OutDataTypeStr=boolean
  Estado del controlador : Outport
  wires:
  [Entrada] -> Operador logico/1, Memoria de pulsacion del joystick/Enable
  Estado del boton/1 -> Memoria de pulsacion del teclado/1(Estado del boton), Memoria de pulsacion del joystick/1(Estado del boton)
  Reinicio/1 -> Memoria de pulsacion del teclado/2(Reinicio), Memoria de pulsacion del joystick/2(Reinicio)
  Operador logico/1 -> Memoria de pulsacion del teclado/Enable
  Memoria de pulsacion del joystick/1(Estado del controlador) -> Operador logico1/1
  Memoria de pulsacion del teclado/1(Estado del controlador) -> Operador logico1/2
  Operador logico1/1 -> Estado del controlador/1

== system Simulador/Autopiloto/Activador de controladores/Interruptor con latch3 ==
  Estado del boton : Inport
  Reinicio : Inport  Port=2
  Memoria de pulsacion del joystick : Subsystem  TreatAsAtomicUnit=on
  Memoria de pulsacion del teclado : Subsystem  TreatAsAtomicUnit=on
  Operador logico : Logic  Operator=NOT  AllPortsSameDT=off  OutDataTypeStr=boolean
  Operador logico1 : Logic  Operator=OR  AllPortsSameDT=off  OutDataTypeStr=boolean
  Estado del controlador : Outport
  wires:
  [Entrada] -> Operador logico/1, Memoria de pulsacion del joystick/Enable
  Estado del boton/1 -> Memoria de pulsacion del teclado/1(Estado del boton), Memoria de pulsacion del joystick/1(Estado del boton)
  Reinicio/1 -> Memoria de pulsacion del teclado/2(Reinicio), Memoria de pulsacion del joystick/2(Reinicio)
  Operador logico/1 -> Memoria de pulsacion del teclado/Enable
  Memoria de pulsacion del joystick/1(Estado del controlador) -> Operador logico1/1
  Memoria de pulsacion del teclado/1(Estado del controlador) -> Operador logico1/2
  Operador logico1/1 -> Estado del controlador/1

== system Simulador/Autopiloto/Activador de controladores/Interruptor con latch4 ==
  Estado del boton : Inport
  Reinicio : Inport  Port=2
  Memoria de pulsacion del joystick : Subsystem  TreatAsAtomicUnit=on
  Memoria de pulsacion del teclado : Subsystem  TreatAsAtomicUnit=on
  Operador logico : Logic  Operator=NOT  AllPortsSameDT=off  OutDataTypeStr=boolean
  Operador logico1 : Logic  Operator=OR  AllPortsSameDT=off  OutDataTypeStr=boolean
  Estado del controlador : Outport
  wires:
  [Entrada] -> Operador logico/1, Memoria de pulsacion del joystick/Enable
  Estado del boton/1 -> Memoria de pulsacion del teclado/1(Estado del boton), Memoria de pulsacion del joystick/1(Estado del boton)
  Reinicio/1 -> Memoria de pulsacion del teclado/2(Reinicio), Memoria de pulsacion del joystick/2(Reinicio)
  Operador logico/1 -> Memoria de pulsacion del teclado/Enable
  Memoria de pulsacion del joystick/1(Estado del controlador) -> Operador logico1/1
  Memoria de pulsacion del teclado/1(Estado del controlador) -> Operador logico1/2
  Operador logico1/1 -> Estado del controlador/1

== system Simulador/Autopiloto/Activador de controladores/Interruptor con latch5 ==
  Estado del boton : Inport
  Reinicio : Inport  Port=2
  Memoria de pulsacion del joystick : Subsystem  TreatAsAtomicUnit=on
  Memoria de pulsacion del teclado : Subsystem  TreatAsAtomicUnit=on
  Operador logico : Logic  Operator=NOT  AllPortsSameDT=off  OutDataTypeStr=boolean
  Operador logico1 : Logic  Operator=OR  AllPortsSameDT=off  OutDataTypeStr=boolean
  Estado del controlador : Outport
  wires:
  [Entrada] -> Operador logico/1, Memoria de pulsacion del joystick/Enable
  Estado del boton/1 -> Memoria de pulsacion del teclado/1(Estado del boton), Memoria de pulsacion del joystick/1(Estado del boton)
  Reinicio/1 -> Memoria de pulsacion del teclado/2(Reinicio), Memoria de pulsacion del joystick/2(Reinicio)
  Operador logico/1 -> Memoria de pulsacion del teclado/Enable
  Memoria de pulsacion del joystick/1(Estado del controlador) -> Operador logico1/1
  Memoria de pulsacion del teclado/1(Estado del controlador) -> Operador logico1/2
  Operador logico1/1 -> Estado del controlador/1

== system Simulador/Autopiloto/Activador de controladores/Interruptor con latch6 ==
  Estado del boton : Inport
  Reinicio : Inport  Port=2
  Memoria de pulsacion del joystick : Subsystem  TreatAsAtomicUnit=on
  Memoria de pulsacion del teclado : Subsystem  TreatAsAtomicUnit=on
  Operador logico : Logic  Operator=NOT  AllPortsSameDT=off  OutDataTypeStr=boolean
  Operador logico1 : Logic  Operator=OR  AllPortsSameDT=off  OutDataTypeStr=boolean
  Estado del controlador : Outport
  wires:
  [Entrada] -> Operador logico/1, Memoria de pulsacion del joystick/Enable
  Estado del boton/1 -> Memoria de pulsacion del teclado/1(Estado del boton), Memoria de pulsacion del joystick/1(Estado del boton)
  Reinicio/1 -> Memoria de pulsacion del teclado/2(Reinicio), Memoria de pulsacion del joystick/2(Reinicio)
  Operador logico/1 -> Memoria de pulsacion del teclado/Enable
  Memoria de pulsacion del joystick/1(Estado del controlador) -> Operador logico1/1
  Memoria de pulsacion del teclado/1(Estado del controlador) -> Operador logico1/2
  Operador logico1/1 -> Estado del controlador/1

== system Simulador/Autopiloto/Activador de controladores/Interruptor con latch7 ==
  Estado del boton : Inport
  Reinicio : Inport  Port=2
  Memoria de pulsacion del joystick : Subsystem  TreatAsAtomicUnit=on
  Memoria de pulsacion del teclado : Subsystem  TreatAsAtomicUnit=on
  Operador logico : Logic  Operator=NOT  AllPortsSameDT=off  OutDataTypeStr=boolean
  Operador logico1 : Logic  Operator=OR  AllPortsSameDT=off  OutDataTypeStr=boolean
  Estado del controlador : Outport
  wires:
  [Entrada] -> Operador logico/1, Memoria de pulsacion del joystick/Enable
  Estado del boton/1 -> Memoria de pulsacion del teclado/1(Estado del boton), Memoria de pulsacion del joystick/1(Estado del boton)
  Reinicio/1 -> Memoria de pulsacion del teclado/2(Reinicio), Memoria de pulsacion del joystick/2(Reinicio)
  Operador logico/1 -> Memoria de pulsacion del teclado/Enable
  Memoria de pulsacion del joystick/1(Estado del controlador) -> Operador logico1/1
  Memoria de pulsacion del teclado/1(Estado del controlador) -> Operador logico1/2
  Operador logico1/1 -> Estado del controlador/1

== system Simulador/Autopiloto/Activador de controladores/Interruptor con latch8 ==
  Estado del boton : Inport
  Reinicio : Inport  Port=2
  Memoria de pulsacion del joystick : Subsystem  TreatAsAtomicUnit=on
  Memoria de pulsacion del teclado : Subsystem  TreatAsAtomicUnit=on
  Operador logico : Logic  Operator=NOT  AllPortsSameDT=off  OutDataTypeStr=boolean
  Operador logico1 : Logic  Operator=OR  AllPortsSameDT=off  OutDataTypeStr=boolean
  Estado del controlador : Outport
  wires:
  [Entrada] -> Operador logico/1, Memoria de pulsacion del joystick/Enable
  Estado del boton/1 -> Memoria de pulsacion del teclado/1(Estado del boton), Memoria de pulsacion del joystick/1(Estado del boton)
  Reinicio/1 -> Memoria de pulsacion del teclado/2(Reinicio), Memoria de pulsacion del joystick/2(Reinicio)
  Operador logico/1 -> Memoria de pulsacion del teclado/Enable
  Memoria de pulsacion del joystick/1(Estado del controlador) -> Operador logico1/1
  Memoria de pulsacion del teclado/1(Estado del controlador) -> Operador logico1/2
  Operador logico1/1 -> Estado del controlador/1

== system Simulador/Autopiloto/Activador de controladores/Interruptor con latch9 ==
  Estado del boton : Inport
  Reinicio : Inport  Port=2
  Memoria de pulsacion del joystick : Subsystem  TreatAsAtomicUnit=on
  Memoria de pulsacion del teclado : Subsystem  TreatAsAtomicUnit=on
  Operador logico : Logic  Operator=NOT  AllPortsSameDT=off  OutDataTypeStr=boolean
  Operador logico1 : Logic  Operator=OR  AllPortsSameDT=off  OutDataTypeStr=boolean
  Estado del controlador : Outport
  wires:
  [Entrada] -> Operador logico/1, Memoria de pulsacion del joystick/Enable
  Estado del boton/1 -> Memoria de pulsacion del teclado/1(Estado del boton), Memoria de pulsacion del joystick/1(Estado del boton)
  Reinicio/1 -> Memoria de pulsacion del teclado/2(Reinicio), Memoria de pulsacion del joystick/2(Reinicio)
  Operador logico/1 -> Memoria de pulsacion del teclado/Enable
  Memoria de pulsacion del joystick/1(Estado del controlador) -> Operador logico1/1
  Memoria de pulsacion del teclado/1(Estado del controlador) -> Operador logico1/2
  Operador logico1/1 -> Estado del controlador/1

== system Simulador/Autopiloto/Calculador de coeficientes aerodinamicos (alpha)/Modulo de Va_total ==
  "Ua, Va, Wa" : Inport
  Al cuadrado : Math  Operator=magnitude^2  SaturateOnIntegerOverflow=on
  Al cuadrado1 : Math  Operator=magnitude^2  SaturateOnIntegerOverflow=on
  Al cuadrado2 : Math  Operator=magnitude^2  SaturateOnIntegerOverflow=on
  Demux1 : Demux  Outputs=3
  Raiz cuadrada : Sqrt  SaturateOnIntegerOverflow=on
  Sum2 : Sum  Inputs=+++
  Va_total : Outport
  wires:
  "Ua, Va, Wa"/1 -> Demux1/1
  Demux1/2 -> Al cuadrado1/1
  Demux1/1 -> Al cuadrado/1
  Demux1/3 -> Al cuadrado2/1
  Al cuadrado1/1 -> Sum2/2
  Al cuadrado2/1 -> Sum2/3
  Al cuadrado/1 -> Sum2/1
  Sum2/1 -> Raiz cuadrada/1
  Raiz cuadrada/1 -> Va_total/1

== system Simulador/Autopiloto/Controlador de Uinf mediante delta_t/Modulo de Va_total ==
  "Ua, Va, Wa" : Inport
  Al cuadrado : Math  Operator=magnitude^2  SaturateOnIntegerOverflow=on
  Al cuadrado1 : Math  Operator=magnitude^2  SaturateOnIntegerOverflow=on
  Al cuadrado2 : Math  Operator=magnitude^2  SaturateOnIntegerOverflow=on
  Demux1 : Demux  Outputs=3
  Raiz cuadrada : Sqrt  SaturateOnIntegerOverflow=on
  Sum2 : Sum  Inputs=+++
  Va_total : Outport
  wires:
  "Ua, Va, Wa"/1 -> Demux1/1
  Demux1/2 -> Al cuadrado1/1
  Demux1/1 -> Al cuadrado/1
  Demux1/3 -> Al cuadrado2/1
  Al cuadrado1/1 -> Sum2/2
  Al cuadrado2/1 -> Sum2/3
  Al cuadrado/1 -> Sum2/1
  Sum2/1 -> Raiz cuadrada/1
  Raiz cuadrada/1 -> Va_total/1

== system Simulador/Autopiloto/Controlador de Uinf mediante theta/Modulo de Va_total ==
  "Ua, Va, Wa" : Inport
  Al cuadrado : Math  Operator=magnitude^2  SaturateOnIntegerOverflow=on
  Al cuadrado1 : Math  Operator=magnitude^2  SaturateOnIntegerOverflow=on
  Al cuadrado2 : Math  Operator=magnitude^2  SaturateOnIntegerOverflow=on
  Demux1 : Demux  Outputs=3
  Raiz cuadrada : Sqrt  SaturateOnIntegerOverflow=on
  Sum2 : Sum  Inputs=+++
  Va_total : Outport
  wires:
  "Ua, Va, Wa"/1 -> Demux1/1
  Demux1/2 -> Al cuadrado1/1
  Demux1/1 -> Al cuadrado/1
  Demux1/3 -> Al cuadrado2/1
  Al cuadrado1/1 -> Sum2/2
  Al cuadrado2/1 -> Sum2/3
  Al cuadrado/1 -> Sum2/1
  Sum2/1 -> Raiz cuadrada/1
  Raiz cuadrada/1 -> Va_total/1

== system Simulador/Autopiloto/Reconocedor de inicio del controlador de psi/Psi de inicio ==
  Psi : Inport
  Disparador : TriggerPort  StatesWhenEnabling=reset  ShowOutputPort=on  PortDimensions=1
  Interruptor : Switch  Criteria=u2 > Threshold
  Tierra : Ground
  Psi_ : Outport
  wires:
  Psi/1 -> Interruptor/1
  Interruptor/1 -> Psi_/1
  Disparador/1 -> Interruptor/2
  Tierra/1 -> Interruptor/3

== system Simulador/Dinamica/Calculador de coeficientes aerodinamicos/Modulo de Va_total ==
  "Ua, Va, Wa" : Inport
  Al cuadrado : Math  Operator=magnitude^2  SaturateOnIntegerOverflow=on
  Al cuadrado1 : Math  Operator=magnitude^2  SaturateOnIntegerOverflow=on
  Al cuadrado2 : Math  Operator=magnitude^2  SaturateOnIntegerOverflow=on
  Demux1 : Demux  Outputs=3
  Raiz cuadrada : Sqrt  SaturateOnIntegerOverflow=on
  Sum2 : Sum  Inputs=+++
  Va_total : Outport
  wires:
  "Ua, Va, Wa"/1 -> Demux1/1
  Demux1/2 -> Al cuadrado1/1
  Demux1/1 -> Al cuadrado/1
  Demux1/3 -> Al cuadrado2/1
  Al cuadrado1/1 -> Sum2/2
  Al cuadrado2/1 -> Sum2/3
  Al cuadrado/1 -> Sum2/1
  Sum2/1 -> Raiz cuadrada/1
  Raiz cuadrada/1 -> Va_total/1

== system Simulador/Entrada de control manual/Teclado/Reconocedor de teclado ==
  Tecla : Inport  PortDimensions=1
  Ejes : Inport  Port=2  PortDimensions=3
  Pulsacion : Inport  Port=3  PortDimensions=1
  Activador : EnablePort
  Demux3 : Demux  Outputs=3
  Interruptor de eventos : SwitchCase  CaseConditions={39,48,49,50,51,52,53,54,55,56,57,[97,100],[115,119],[102,114]}
  Mux : Mux  Inputs=3
  Mux1 : Mux  Inputs=11
  Subsistema de accion del interruptor de eventos : Subsystem  TreatAsAtomicUnit=on
  Subsistema de accion del interruptor de eventos1 : Subsystem  TreatAsAtomicUnit=on
  Subsistema de accion del interruptor de eventos10 : Subsystem  TreatAsAtomicUnit=on
  Subsistema de accion del interruptor de eventos11 : Subsystem  TreatAsAtomicUnit=on
  Subsistema de accion del interruptor de eventos12 : Subsystem  TreatAsAtomicUnit=on
  Subsistema de accion del interruptor de eventos13 : Subsystem  TreatAsAtomicUnit=on
  Subsistema de accion del interruptor de eventos2 : Subsystem  TreatAsAtomicUnit=on
  Subsistema de accion del interruptor de eventos3 : Subsystem  TreatAsAtomicUnit=on
  Subsistema de accion del interruptor de eventos4 : Subsystem  TreatAsAtomicUnit=on
  Subsistema de accion del interruptor de eventos5 : Subsystem  TreatAsAtomicUnit=on
  Subsistema de accion del interruptor de eventos6 : Subsystem  TreatAsAtomicUnit=on
  Subsistema de accion del interruptor de eventos7 : Subsystem  TreatAsAtomicUnit=on
  Subsistema de accion del interruptor de eventos8 : Subsystem  TreatAsAtomicUnit=on
  Subsistema de accion del interruptor de eventos9 : Subsystem  TreatAsAtomicUnit=on
  Terminador : Terminator
  Ejes_ : Outport  PortDimensions=3
  Botones_ : Outport  Port=2  PortDimensions=11
  wires:
  Tecla/1 -> Subsistema de accion del interruptor de eventos/2(Tecla), Subsistema de accion del interruptor de eventos1/2(Tecla), Subsistema de accion del interruptor de eventos2/2(Tecla), Interruptor de eventos/1
  Ejes/1 -> Demux3/1
  Interruptor de eventos/15 -> Terminador/1
  Demux3/2 -> Subsistema de accion del interruptor de eventos1/1(Eje elevadores)
  Subsistema de accion del interruptor de eventos1/1(Eje elevadores_) -> Mux/2
  Demux3/1 -> Subsistema de accion del interruptor de eventos/1(Eje alerones)
  Demux3/3 -> Subsistema de accion del interruptor de eventos2/1(Eje motor)
  Subsistema de accion del interruptor de eventos/1(Eje alerones_) -> Mux/1
  Subsistema de accion del interruptor de eventos2/1(Eje motor_) -> Mux/3
  Mux/1 -> Ejes_/1
  Pulsacion/1 -> Subsistema de accion del interruptor de eventos4/1(Pulsacion), Subsistema de accion del interruptor de eventos5/1(Pulsacion), Subsistema de accion del interruptor de eventos6/1(Pulsacion), Subsistema de accion del interruptor de eventos7/1(Pulsacion), Subsistema de accion del interruptor de eventos8/1(Pulsacion), Subsistema de accion del interruptor de eventos9/1(Pulsacion), Subsistema de accion del interruptor de eventos10/1(Pulsacion), Subsistema de accion del interruptor de eventos11/1(Pulsacion), Subsistema de accion del interruptor de eventos13/1(Pulsacion), Subsistema de accion del interruptor de eventos12/1(Pulsacion), Subsistema de accion del interruptor de eventos3/1(Pulsacion)
  Subsistema de accion del interruptor de eventos3/1(Boton_) -> Mux1/1
  Subsistema de accion del interruptor de eventos13/1(Boton_) -> Mux1/11
  Subsistema de accion del interruptor de eventos12/1(Boton_) -> Mux1/10
  Subsistema de accion del interruptor de eventos11/1(Boton_) -> Mux1/9
  Subsistema de accion del interruptor de eventos10/1(Boton_) -> Mux1/8
  Subsistema de accion del interruptor de eventos9/1(Boton_) -> Mux1/7
  Subsistema de accion del interruptor de eventos8/1(Boton_) -> Mux1/6
  Subsistema de accion del interruptor de eventos7/1(Boton_) -> Mux1/5
  Subsistema de accion del interruptor de eventos6/1(Boton_) -> Mux1/4
  Subsistema de accion del interruptor de eventos5/1(Boton_) -> Mux1/3
  Subsistema de accion del interruptor de eventos4/1(Boton_) -> Mux1/2
  Mux1/1 -> Botones_/1
  Interruptor de eventos/1 -> Subsistema de accion del interruptor de eventos3/Action
  Interruptor de eventos/2 -> Subsistema de accion del interruptor de eventos7/Action
  Interruptor de eventos/3 -> Subsistema de accion del interruptor de eventos8/Action
  Interruptor de eventos/4 -> Subsistema de accion del interruptor de eventos9/Action
  Interruptor de eventos/5 -> Subsistema de accion del interruptor de eventos10/Action
  Interruptor de eventos/6 -> Subsistema de accion del interruptor de eventos11/Action
  Interruptor de eventos/7 -> Subsistema de accion del interruptor de eventos12/Action
  Interruptor de eventos/8 -> Subsistema de accion del interruptor de eventos13/Action
  Interruptor de eventos/9 -> Subsistema de accion del interruptor de eventos4/Action
  Interruptor de eventos/10 -> Subsistema de accion del interruptor de eventos5/Action
  Interruptor de eventos/11 -> Subsistema de accion del interruptor de eventos6/Action
  Interruptor de eventos/12 -> Subsistema de accion del interruptor de eventos/Action
  Interruptor de eventos/13 -> Subsistema de accion del interruptor de eventos1/Action
  Interruptor de eventos/14 -> Subsistema de accion del interruptor de eventos2/Action

== system Simulador/Mision/Gestor de GPS/Envio de datos ==
  Datos : Inport
  Activador : EnablePort
  Envio mediante protocolo UDP : instrumentlib/UDP Send  Host=localhost  Port=3333  LocalPort=3334  EnableBlockingMode=on  ByteOrder=BigEndian
  wires:
  Datos/1 -> Envio mediante protocolo UDP/1

== system Simulador/Mision/Reconocedor de reinicio de FMS/Posicion_NED de reinicio ==
  Posicion_NED : Inport
  Disparador : TriggerPort  StatesWhenEnabling=reset  ShowOutputPort=on  PortDimensions=1
  Interruptor : Switch  Criteria=u2 > Threshold
  Tierra : Ground
  Posicion_NED_ : Outport
  wires:
  Posicion_NED/1 -> Interruptor/1
  Interruptor/1 -> Posicion_NED_/1
  Disparador/1 -> Interruptor/2
  Tierra/1 -> Interruptor/3

== system Simulador/Autopiloto/Activador de controladores/Interruptor con latch/Memoria de pulsacion del joystick ==
  Estado del boton : Inport
  Reinicio : Inport  Port=2
  Activador : EnablePort
  Interruptor1 : Switch  Criteria=u2 > Threshold
  Interruptor2 : Switch  Criteria=u2 > Threshold
  Latch D : simulink_extras/Flip Flops/D Latch
  Operador logico : Logic  Operator=NOT  AllPortsSameDT=off  OutDataTypeStr=boolean
  Operador logico1 : Logic  Operator=NOT  AllPortsSameDT=off  OutDataTypeStr=boolean
  Operador logico2 : Logic  Operator=XOR  AllPortsSameDT=off  OutDataTypeStr=boolean
  Retraso : Delay  DelayLength=1  InitialCondition=0  SampleTime=0.5
  Terminador : Terminator
  Estado del controlador : Outport
  wires:
  Latch D/2 -> Terminador/1
  Latch D/1 -> Retraso/1, Estado del controlador/1
  Operador logico/1 -> Interruptor1/1
  Retraso/1 -> Interruptor1/2
  Estado del boton/1 -> Operador logico/1, Interruptor1/3, Operador logico2/1
  Interruptor2/1 -> Latch D/1
  Interruptor1/1 -> Interruptor2/3
  Operador logico1/1 -> Interruptor2/1
  Operador logico2/1 -> Latch D/2
  Reinicio/1 -> Interruptor2/2, Operador logico1/1, Operador logico2/2
